simulink model "prob1"  (R2020a)
settings: Solver=VariableStepAuto  StartTime=0.0  StopTime=10.0  RelTol=1e-3
settings Model: Creator=vijay  LastModifiedBy=vijay

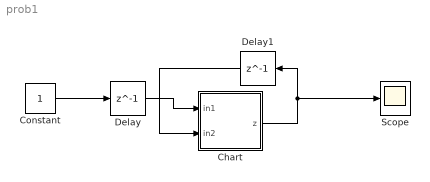
== system prob1 ==
  Chart : Stateflow chart  TreatAsAtomicUnit=on
  Constant : Constant
  Delay : Delay  DelayLength=1
  Delay1 : Delay  DelayLength=1
  Scope : Scope
  wires:
  Constant/1 -> Delay/1
  Chart/1(z) -> Delay1/1, Scope/1
  Delay/1 -> Chart/1(in1)
  Delay1/1 -> Chart/2(in2)

== stateflow chart prob1/Chart ==
  state counter
    entry:
    x=in1;
    y=in2;
    z=x+y;
  state counter1
    entry:
    z=0;
    exit:
    z=x+y;
  counter -> counter [order 2] : [z<4]
  (default) -> counter
  counter1 -> counter1 [order 1] : [z>=4]
  counter -> counter1 [order 1] : [z>=4]
  counter1 -> counter [order 2] : [z<4]
  data: x local; y local; in1 input; in2 input; z output
